simulink model "design_ctrl_imu_yaw"  (R2013b)
settings: Solver=ode45  StartTime=0.0  StopTime=20  FixedStep=0.01  MaxStep=1e-3  MinStep=1e-5  RelTol=1e-3
PreLoadFcn:
  | load('imu_yaw');
libraries: simulink x1, slident x1
settings Model: Creator=Ugo Pattacini  LastModifiedBy=Ugo Pattacini
settings GRTTargetCC: CodeReplacementLibrary=C89/C90 (ANSI)

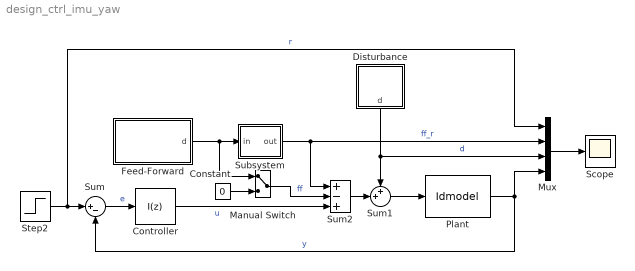
== system design_ctrl_imu_yaw ==
  Constant : Constant  Value=0
  Controller : simulink/Continuous/PID Controller  Controller=I  TimeDomain=Discrete-time  SampleTime=0.01  IntegratorMethod=Trapezoidal  FilterMethod=Trapezoidal  Form=Parallel  P=0  I=11  D=0  N=100  InitialConditionSource=internal  InitialConditionForIntegrator=0  InitialConditionForFilter=0  ExternalReset=none  LimitOutput=off  UpperSaturationLimit=inf  LowerSaturationLimit=-inf  LinearizeAsGain=off  AntiWindupMode=none  Kb=1  TrackingMode=off  Kt=1  PParamMin=[]  PParamMax=[]  IParamMin=[]  IParamMax=[]  DParamMin=[]  DParamMax=[]  NParamMin=[]  NParamMax=[]  KbParamMin=[]  KbParamMax=[]  KtParamMin=[]  KtParamMax=[]  POutMin=[]  POutMax=[]  IOutMin=[]  IOutMax=[]  DOutMin=[]  DOutMax=[]  NOutMin=[]  NOutMax=[]  KbOutMin=[]  KbOutMax=[]  KtOutMin=[]  KtOutMax=[]  IntegratorOutMin=[]  IntegratorOutMax=[]  FilterOutMin=[]  FilterOutMax=[]  SumOutMin=[]  SumOutMax=[]  SumI1OutMin=[]  SumI1OutMax=[]  SumI2OutMin=[]  SumI2OutMax=[]  SumI3OutMin=[]  SumI3OutMax=[]  SumDOutMin=[]  SumDOutMax=[]  SaturationOutMin=[]  SaturationOutMax=[]  IntegratorContinuousStateAttributes=''  IntegratorStateMustResolveToSignalObject=off  IntegratorRTWStateStorageClass=Auto  FilterContinuousStateAttributes=''  FilterStateMustResolveToSignalObject=off  FilterRTWStateStorageClass=Auto  DifferentiatorICPrevScaledInput=0  DifferentiatorOutMin=[]  DifferentiatorOutMax=[]  UseFilter=on
  Disturbance : Subsystem  mask{A=2, t0=4, T=10}
      mask prompts: A "Amplitude"; t0 "Trigger time [s]"; T "Duration [s]"
      mask Display: disp(sprintf('A=%g\nt0=%g\nT=%g',A,t0,T));
  Feed-Forward : Subsystem  mask{A=5, t0=7, T=5}
      mask prompts: A "Amplitude"; t0 "Trigger time [s]"; T "Duration [s]"
      mask Display: disp(sprintf('A=%g\nt0=%g\nT=%g',A,t0,T));
  Manual Switch : ManualSwitch
  Mux : Mux
  "Plant " : slident/Models/Idmodel  sys=imu_yaw  IC=0  noi=off  seed=[]
  Scope : Scope
      settings: ShowLegends=on
  Step2 : Step  Time=5  After=10  SampleTime=0
  Subsystem : Subsystem
  Sum : Sum  Inputs=|+-
  Sum1 : Sum  Inputs=++|
  Sum2 : Sum  Inputs=+-+
  wires:
  Step2/1 -> Mux/1, Sum/1  "r"
  "Plant "/1 -> Mux/4, Sum/2  "y"
  Sum/1 -> Controller/1  "e"
  Sum1/1 -> "Plant "/1
  Mux/1 -> Scope/1
  Controller/1 -> Sum2/3  "u"
  Sum2/1 -> Sum1/2
  Feed-Forward/1(d) -> Manual Switch/1, Subsystem/1(in)
  Manual Switch/1 -> Sum2/2  "ff"
  Constant/1 -> Manual Switch/2
  Disturbance/1(d) -> Sum1/1, Mux/3  "d"
  Subsystem/1(out) -> Sum2/1, Mux/2  "ff_r"

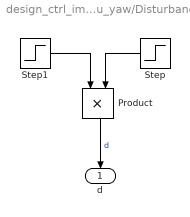
== system design_ctrl_imu_yaw/Disturbance ==
  Product : Product
  Step : Step  Time=t0  After=A  SampleTime=0
  Step1 : Step  Time=t0+T  Before=A  After=0  SampleTime=0
  d : Outport
  wires:
  Step/1 -> Product/2
  Product/1 -> d/1  "d"
  Step1/1 -> Product/1

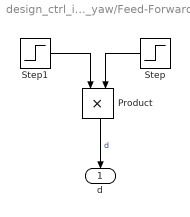
== system design_ctrl_imu_yaw/Feed-Forward ==
  Product : Product
  Step : Step  Time=t0  After=A  SampleTime=0
  Step1 : Step  Time=t0+T  Before=A  After=0  SampleTime=0
  d : Outport
  wires:
  Step1/1 -> Product/1
  Product/1 -> d/1  "d"
  Step/1 -> Product/2

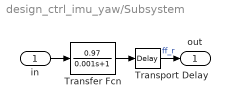
== system design_ctrl_imu_yaw/Subsystem ==
  in : Inport
  Transfer Fcn : TransferFcn  Numerator=[0.97]  Denominator=[0.001 1]
  Transport Delay : TransportDelay  DelayTime=0.01
  out : Outport
  wires:
  in/1 -> Transfer Fcn/1
  Transport Delay/1 -> out/1  "ff_r"
  Transfer Fcn/1 -> Transport Delay/1
